simulink model "doc_gmskintro"  (R2014a)
settings: Solver=FixedStepDiscrete  StartTime=0.0  StopTime=2000.0  RelTol=1e-3
undefined symbols (not defined in the file or in its folder): rsgenpoly
libraries: commblkcod2 x2, commsink2 x2, commdigbbndcpm2 x2, commcnvintrlv2 x2, commchan3 x1, commrandsrc2 x1, dspsigops x1, simulink x1
settings Model: CovMetricSettings=d  Creator=The MathWorks Inc.
settings DataIOCC: SignalLoggingSaveFormat=ModelDataLogs  SignalLoggingName=logsOut
settings OptimizationCC: BlockReduction=off  BooleanDataType=off  ExpressionDepthLimit=2147483647
settings DebuggingCC: SaveWithParameterizedLinksMsg=none  UnderspecifiedInitializationDetection=Classic  SignalResolutionControl=TryResolveAllWithWarning  SolverPrmCheckMsg=none  MultiTaskDSMMsg=warning  MultiTaskCondExecSysMsg=none  FcnCallInpInsideContextMsg=UseLocalSettings  StateNameClashWarn=warning  StrictBusMsg=None
settings HardwareCC: TargetUnknown=on
settings RTWCC: IncludeERTFirstTime=on
settings GRTTargetCC: TargetFcnLib=iso_c_tmw.mat  CombineOutputUpdateFcns=off  GRTInterface=on

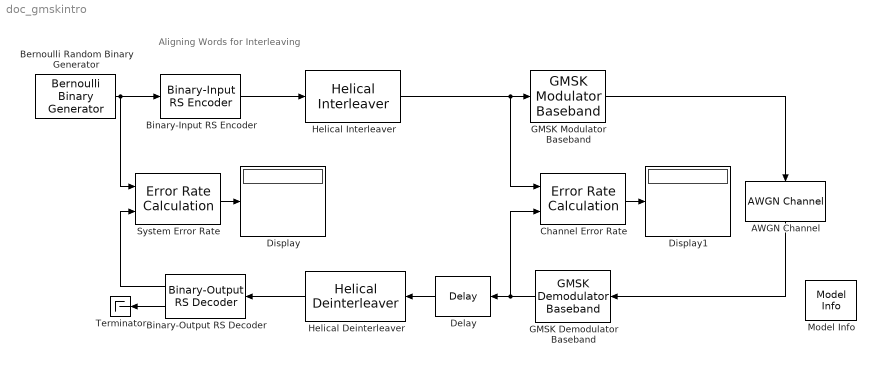
== system doc_gmskintro ==
  note: Aligning Words for Interleaving
  AWGN Channel : commchan3/AWGN Channel  InputProcessing=Columns as channels (frame based)  seed=18233  noiseMode="Signal to noise ratio  (SNR)"  EbNodB=10  EsNodB=50  SNRdB=-6  bitsPerSym=1  Ps=1  Tsym=12  variance=1
  Bernoulli Random Binary Generator : commrandsrc2/Bernoulli Binary Generator  P=.5  seed=0  Ts=.1  frameBased=on  sampPerFrame=15  orient=off  outDataType=double
  Binary-Input RS Encoder : commblkcod2/Binary-Input RS Encoder  n=7  k=5  specPrimPoly=off  prPoly=[1 0 1 1]  specGenPoly=off  genPoly=rsgenpoly(7,3)  specPuncture=off  punctVec=[ones(2,1); zeros(2,1)]  outDType=Same as input
  Binary-Output RS Decoder : commblkcod2/Binary-Output RS Decoder  n=7  k=5  specPrimPoly=off  prPoly=[1 0 1 1]  specGenPoly=off  genPoly=rsgenpoly(7,3)  specPuncture=off  punctVec=[ones(2,1); zeros(2,1)]  specErasurePort=off  showNumErr=on  outDType=Same as input
  Channel Error Rate : commsink2/Error Rate Calculation  N=16  st_delay=0  cp_mode=Entire frame  subframe=[]  PMode=Port  WsName=ErrorVec  RsMode2=off  stop=off  numErr=100  maxBits=1000
  Delay : dspsigops/Delay  InputProcessing=Columns as channels (frame based)  dly_unit=Samples  delay=5  ic_detail=off  dif_ic_for_ch=off  dif_ic_for_dly=off  ic=0  reset_popup=None
  Display : Display
  Display1 : Display
  GMSK Demodulator Baseband : commdigbbndcpm2/GMSK Demodulator Baseband  OutputType=Bit  BT=.3  pulseLength=3  preHistory=1  phaseOffset=0  samplesPerSymbol=16  RateOptions=Enforce single-rate processing  traceBack=16  outDType=double
  GMSK Modulator Baseband : commdigbbndcpm2/GMSK Modulator Baseband  inputType=Bit  BT=.3  pulseLength=3  preHistory=1  phaseOffset=0  samplesPerSymbol=16  RateOptions=Enforce single-rate processing  outDataType=double
  Helical Deinterleaver : commcnvintrlv2/Helical Deinterleaver  C=7  N=3  s=1  ic=0
  Helical Interleaver : commcnvintrlv2/Helical Interleaver  C=7  N=3  s=1  ic=0
  Model Info : simulink/Model-Wide Utilities/Model Info  InitialBlockCM=None  BlockCM=none  Frame=on  DisplayStringWithTags=Info  HorizontalTextAlignment=Center  LeftAlignmentValue=0.5  SourceBlockDiagram=doc_gmskintro  TagMaxNumber=20
  System Error Rate : commsink2/Error Rate Calculation  N=15*3  st_delay=0  cp_mode=Entire frame  subframe=[]  PMode=Port  WsName=ErrorVec  RsMode2=off  stop=off  numErr=100  maxBits=1000
  Terminator : Terminator
  wires:
  GMSK Modulator Baseband/1 -> AWGN Channel/1
  System Error Rate/1 -> Display/1
  AWGN Channel/1 -> GMSK Demodulator Baseband/1
  Bernoulli Random Binary Generator/1 -> System Error Rate/1, Binary-Input RS Encoder/1
  Delay/1 -> Helical Deinterleaver/1
  Helical Interleaver/1 -> Channel Error Rate/1, GMSK Modulator Baseband/1
  GMSK Demodulator Baseband/1 -> Channel Error Rate/2, Delay/1
  Binary-Input RS Encoder/1 -> Helical Interleaver/1
  Helical Deinterleaver/1 -> Binary-Output RS Decoder/1
  Binary-Output RS Decoder/1 -> System Error Rate/2
  Binary-Output RS Decoder/2 -> Terminator/1
  Channel Error Rate/1 -> Display1/1
